simulink model "pend_model"  (R2018a)
settings: Solver=FixedStepAuto  StartTime=0.0  StopTime=50  FixedStep=0.005  RelTol=1e-3
values from neighbouring files (symbols this model uses):
  a = (sqrt(ax*ax+ay*ay+az*az))    [Vatli1.m]
  b = cross(v0,B)    [Vatli1.m]
undefined symbols (not defined in the file or in its folder): c, c2, d, f, h, phi111, phi222
settings Model: Creator=DELL  LastModifiedBy=DELL

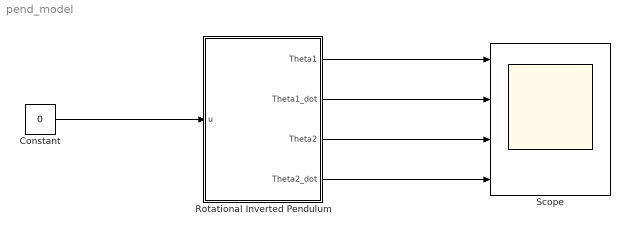
== system pend_model ==
  Constant : Constant  Value=0
  Rotational Inverted Pendulum : Subsystem
  Scope : Scope  NumInputPorts=4
  wires:
  Rotational Inverted Pendulum/1(Theta1) -> Scope/1
  Rotational Inverted Pendulum/2(Theta1_dot) -> Scope/2
  Rotational Inverted Pendulum/3(Theta2) -> Scope/3
  Rotational Inverted Pendulum/4(Theta2_dot) -> Scope/4
  Constant/1 -> Rotational Inverted Pendulum/1(u)

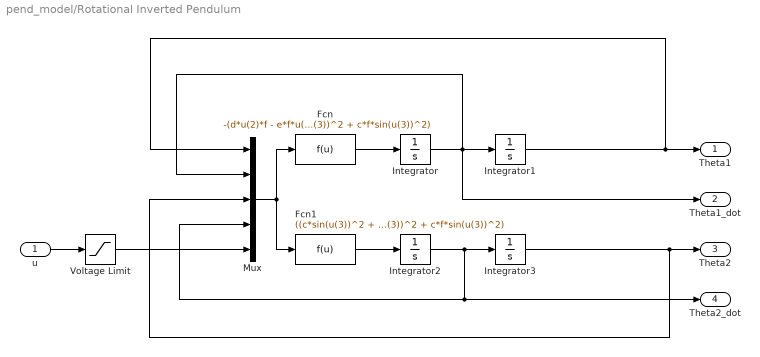
== system pend_model/Rotational Inverted Pendulum ==
  u : Inport
  Fcn : Fcn  Expr=-(d*u(2)*f - e*f*u(5) + b*c2*u(4)*cos(u(3)) + b*u(4)^2*f*sin(u(3)) - b*h*cos(u(3))*sin(u(3)) - b*c*u(2)^2*cos(u(3))^2*sin(u(3)) + 2*c*u(2)*u(4)*f*cos(u(3))*sin(u(3)))/(a*f - b^2*cos(u(3))^2 + c*f*sin(u(3))^2)
  Fcn1 : Fcn  Expr=((c*sin(u(3))^2 + a)*((c*sin(2*u(3))*u(2)^2)/2 - c2*u(4) + h*sin(u(3))))/(a*f - b^2*cos(u(3))^2 + c*f*sin(u(3))^2) - (b*cos(u(3))*(b*sin(u(3))*u(4)^2 + c*u(2)*sin(2*u(3))*u(4) + d*u(2) - e*u(5)))/(a*f - b^2*cos(u(3))^2 + c*f*sin(u(3))^2)
  Integrator : Integrator
  Integrator1 : Integrator  InitialCondition=phi111
  Integrator2 : Integrator
  Integrator3 : Integrator  InitialCondition=phi222
  Mux : Mux  Inputs=5
  "Voltage Limit " : Saturate  UpperLimit=25  LowerLimit=-25
  Theta1 : Outport
  Theta1_dot : Outport  Port=2
  Theta2 : Outport  Port=3
  Theta2_dot : Outport  Port=4
  wires:
  Fcn1/1 -> Integrator2/1
  Fcn/1 -> Integrator/1
  Integrator/1 -> Mux/2, Integrator1/1, Theta1_dot/1
  Integrator2/1 -> Theta2_dot/1, Mux/4, Integrator3/1
  Mux/1 -> Fcn1/1, Fcn/1
  Integrator1/1 -> Mux/1, Theta1/1
  Integrator3/1 -> Mux/3, Theta2/1
  "Voltage Limit "/1 -> Mux/5
  u/1 -> "Voltage Limit "/1
